simulink model "PanelsInSeriesBB_PI"  (R2016a)
settings: Solver=ode23t  StartTime=0.0  StopTime=30  FixedStep=t_PWM/10  MaxStep=2e-6  RelTol=2e-4
values from neighbouring files (symbols this model uses):
  C1 = t_PWM * (N*Impp)*0.1/ (8 * (N*Vmpp)*0.0001)    [SolarPanelModel.m]
  C2 = (N*Vo) * t_PWM/ (Load * (N*Vo)*0.001)    [SolarPanelModel.m]
  delta_Il = (N*Impp)*0.1/ 2    [SolarPanelModel.m]
  G = 1000    [SolarPanelModel.m]
  Gr = 1000    [SolarPanelModel.m]
  Isc = G/ Gr * (Iscr + miu_Isc*(Tc - Tr))    (= 9.318625)    [SolarPanelModel.m]
  Iscr = 9.19    [SolarPanelModel.m]
  K = 1.38 * 10^(-23)    (= 1.38e-23)    [SolarPanelModel.m]
  L_inductor = (N*Vo) * t_PWM/ (4 * (N*Impp)*0.01)    [SolarPanelModel.m]
  m = sol(1)    [SolarPanelModel.m]
  miu_Isc = 0.0049    [SolarPanelModel.m]
  miu_Voc = -0.1184    [SolarPanelModel.m]
  N = 3    [SolarPanelModel.m]
  NOCT = 45    [SolarPanelModel.m]
  q = 1.6 * 10^(-19)    (= 1.6e-19)    [SolarPanelModel.m]
  Rs = sol(3)    [SolarPanelModel.m]
  Rsh = sol(2)    [SolarPanelModel.m]
  T = 273.15    [SolarPanelModel.m]
  t_PWM = 20e-6    (= 2e-05)    [SolarPanelModel.m]
  ta = 20    [SolarPanelModel.m]
  Tr = T + 25    (= 298.15)    [SolarPanelModel.m]
  Vo = 50    [SolarPanelModel.m]
  Voc = Vocr + miu_Voc*(Tc - Tr) + m*Vt*log(G/Gr)    [SolarPanelModel.m]
  Vocr = 38.2    [SolarPanelModel.m]
undefined symbols (not defined in the file or in its folder): Cdc_inv, delta_Ii, g1, k2, kI, kv_ig, Li, Tpv, Tzv
libraries: powerlib x59, simulink x9, powerlib_extras x2, powerlib_meascontrol x1
settings Model: Creator=frede  LastModifiedBy=frede
settings DataIOCC: LimitDataPoints=on  SaveFormat=Array
settings HardwareCC: ProdBitPerPointer=32  ProdLargestAtomicFloat=None  ProdIntDivRoundTo=Undefined  ProdEndianess=Unspecified  ProdWordSize=32  ProdHWDeviceType=32-bit Generic
settings ModelReferenceCC: PropagateSignalLabelsOutOfModel=off
settings ConfigComp: CovModelRefEnable=Off

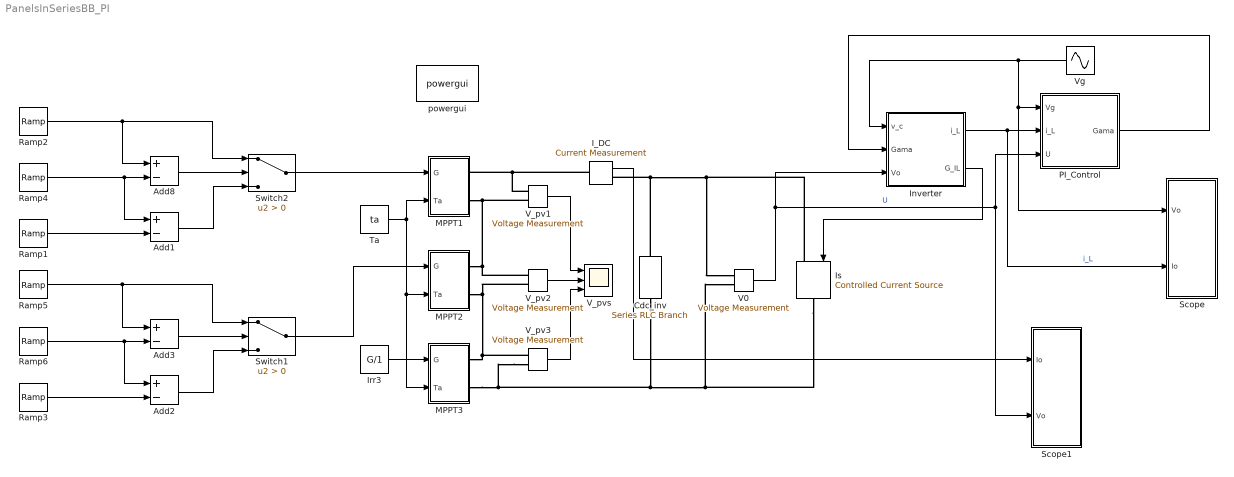
== system PanelsInSeriesBB_PI ==
  Add{1..3,8} (4 alike) : Sum  Inputs=+-
  Cdc_inv : powerlib/Elements/Series RLC Branch  LConnTagsString=__new0  RConnTagsString=__new0  BranchType=RC  Resistance=0.01  Inductance=1e-3  SetiL0=off  InitialCurrent=0  Capacitance=Cdc_inv  Setx0=on  InitialVoltage=Vo  Measurements=None
  I_DC : powerlib/Measurements/Current Measurement  PhasorSimulation=off  OutputType=Complex  PSBequivalent=0
  Inverter : Subsystem
  Irr3 : Constant  Value=G/1
  Is : powerlib/Electrical Sources/Controlled Current Source  Initialize=on  Source_Type=DC  Amplitude=0  Phase=0  Frequency=0  Measurements=None
  MPPT1 : Subsystem
  MPPT2 : Subsystem
  MPPT3 : Subsystem
  PI_Control : Subsystem
  Ramp1 : simulink/Sources/Ramp  slope=31.25  start=t5  X0=0
  Ramp2 : simulink/Sources/Ramp  slope=-31.25  start=t1  X0=g1
  Ramp3 : simulink/Sources/Ramp  slope=25  start=t6  X0=0
  Ramp4 : simulink/Sources/Ramp  slope=31.25  start=-10  X0=0
  Ramp5 : simulink/Sources/Ramp  slope=-25  start=t4  X0=g1
  Ramp6 : simulink/Sources/Ramp  slope=25  start=-20  X0=0
  Scope : Subsystem
  Scope1 : Subsystem
  Switch1 : Switch  Criteria=u2 > Threshold
  Switch2 : Switch  Criteria=u2 > Threshold
  Ta : Constant  Value=ta
  V0 : powerlib/Measurements/Voltage Measurement  PhasorSimulation=off  OutputType=Complex  PSBequivalent=0
  V_pv1 : powerlib/Measurements/Voltage Measurement  PhasorSimulation=off  OutputType=Complex  PSBequivalent=0
  V_pv2 : powerlib/Measurements/Voltage Measurement  PhasorSimulation=off  OutputType=Complex  PSBequivalent=0
  V_pv3 : powerlib/Measurements/Voltage Measurement  PhasorSimulation=off  OutputType=Complex  PSBequivalent=0
  V_pvs : Scope  NumInputPorts=3
  Vg : Sin  Amplitude=sqrt(2)*230  Frequency=2*pi*50  SampleTime=0
  powergui : powerlib/powergui  Priority=1  SimulationMode=Discrete  SolverType=Tustin/Backward Euler (TBE)  SampleTime=t_PWM/10  frequency=60  SPID=off  DisableSnubberDevices=off  DisableRonSwitches=off  DisableVfSwitches=off  SwTol=0  DisplayEquations=off  Interpol=off  ExternalGateDelay=off  methode=off  Ts=10  FunctionMessages=off  echomessages=off  HookPort=off  EnableUseOfTLC=off  x0status=blocks  frequencyindice=0  Pbase=100e6  ErrMax=1e-4  Iterations=50  UnitsV=kV  UnitsW=MW  buscounter=0  RestoreLinks=warning  ResistiveCurrentMeasurement=off  Frange=[0:2:500]  Ylog=off  Xlog=on  ShowGrid=off  save=off  variable=ZData  structure=0  ZoomFFT=off  StartTime=0.0  cycles=1  DisplayStyle=1  fundamental=60  FreqAxis=off  MaxFrequency=1000  frequencyindicesteady=1  RmsSteady=1  display=off
  wires:
  V_pv1/1 -> V_pvs/1
  V_pv2/1 -> V_pvs/2
  V_pv3/1 -> V_pvs/3
  Ta/1 -> MPPT1/2(Ta), MPPT3/2(Ta), MPPT2/2(Ta)
  Irr3/1 -> MPPT3/1(G)
  Switch2/1 -> MPPT1/1(G)
  Switch1/1 -> MPPT2/1(G)
  Vg/1 -> Inverter/1(v_c), Scope/1(Vo), PI_Control/1(Vg)
  PI_Control/1(Gama) -> Inverter/2(Gama)
  Inverter/1(i_L) -> Scope/2(Io), PI_Control/2(i_L)  "i_L"
  V0/1 -> Inverter/3(Vo), PI_Control/3(U), Scope1/2(Vo)  "U"
  Inverter/2(G_IL) -> Is/1
  I_DC/1 -> Scope1/1(Io)
  Ramp4/1 -> Add1/1, Add8/2
  Ramp2/1 -> Switch2/1, Add8/1
  Add8/1 -> Switch2/2
  Ramp1/1 -> Add1/2
  Add1/1 -> Switch2/3
  Ramp6/1 -> Add2/1, Add3/2
  Ramp5/1 -> Switch1/1, Add3/1
  Add3/1 -> Switch1/2
  Ramp3/1 -> Add2/2
  Add2/1 -> Switch1/3
  connections:
  V_pv2/LConn1 -- V_pv1/LConn2 -- MPPT1/RConn2 -- MPPT2/RConn1
  V_pv3/LConn1 -- MPPT3/RConn1 -- V_pv2/LConn2 -- MPPT2/RConn2
  I_DC/LConn1 -- V_pv1/LConn1 -- MPPT1/RConn1
  V_pv3/LConn2 -- Is/RConn1 -- V0/LConn2 -- Cdc_inv/RConn1 -- MPPT3/RConn2
  Cdc_inv/LConn1 -- Is/LConn1 -- V0/LConn1 -- I_DC/RConn1

== system PanelsInSeriesBB_PI/Inverter ==
  v_c : Inport
  Gama : Inport  Port=2
  Vo : Inport  Port=3
  Add1 : Sum  Inputs=+-
  Product : Product
  Product1 : Product
  Transfer Fcn : TransferFcn  Denominator=[Li 3]
  i_L : Outport
  G_IL : Outport  Port=2
  wires:
  Transfer Fcn/1 -> i_L/1, Product/2
  Add1/1 -> Transfer Fcn/1
  Product/1 -> G_IL/1
  Product1/1 -> Add1/1
  v_c/1 -> Add1/2
  Gama/1 -> Product1/2, Product/1
  Vo/1 -> Product1/1

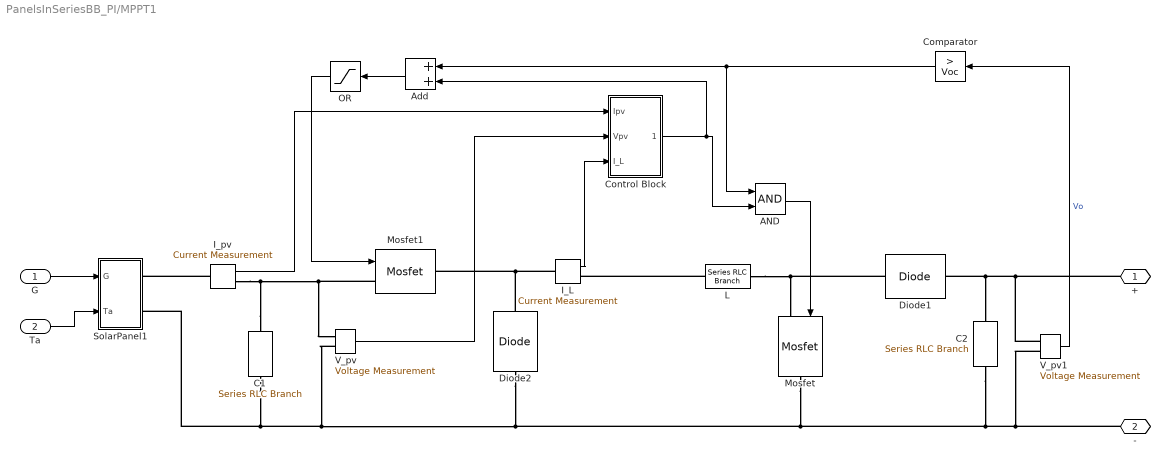
== system PanelsInSeriesBB_PI/MPPT1 ==
  G : Inport
  Ta : Inport  Port=2
  AND : Logic  AllPortsSameDT=off  OutDataTypeStr=boolean
  Add : Sum
  C1 : powerlib/Elements/Series RLC Branch  LConnTagsString=__new0  RConnTagsString=__new0  BranchType=C  Resistance=Rs  Inductance=1e-3  SetiL0=off  InitialCurrent=0  Capacitance=C1  Setx0=on  InitialVoltage=Vmpp  Measurements=None
  C2 : powerlib/Elements/Series RLC Branch  LConnTagsString=__new0  RConnTagsString=__new0  BranchType=C  Resistance=Rs  Inductance=1e-3  SetiL0=off  InitialCurrent=0  Capacitance=C2  Setx0=on  InitialVoltage=Vo/3  Measurements=None
  Comparator : simulink/Logic and Bit Operations/Compare To Constant  relop=>  const=Voc  OutDataTypeStr=boolean
  Control Block : Subsystem
  Diode1 : powerlib/Power Electronics/Diode  Ron=0.001  Lon=0  Vf=0.001  IC=0  UseSnubber=off  Rs=500  Cs=1e-9  Measurements=off
  Diode2 : powerlib/Power Electronics/Diode  Ron=0.001  Lon=0  Vf=0.001  IC=0  UseSnubber=off  Rs=500  Cs=1e-9  Measurements=off
  I_L : powerlib/Measurements/Current Measurement  PhasorSimulation=off  OutputType=Complex  PSBequivalent=0
  I_pv : powerlib/Measurements/Current Measurement  PhasorSimulation=off  OutputType=Complex  PSBequivalent=0
  L : powerlib/Elements/Series RLC Branch  LConnTagsString=__new0  RConnTagsString=__new0  BranchType=L  Resistance=Rs  Inductance=L_inductor  SetiL0=off  InitialCurrent=0  Capacitance=1e-6  Setx0=off  InitialVoltage=0  Measurements=None
  Mosfet : powerlib/Power Electronics/Mosfet  Ron=0.001  Lon=0  Rd=0.001  Vfd=0  IC=0  Rs=1e3  Cs=1e-9  Measurements=off
  Mosfet1 : powerlib/Power Electronics/Mosfet  Ron=0.001  Lon=0  Rd=0.001  Vfd=0  IC=0  Rs=1e3  Cs=1e-9  Measurements=off
  OR : Saturate  UpperLimit=1  LowerLimit=0
  SolarPanel1 : Subsystem
  V_pv : powerlib/Measurements/Voltage Measurement  PhasorSimulation=off  OutputType=Complex  PSBequivalent=0
  V_pv1 : powerlib/Measurements/Voltage Measurement  PhasorSimulation=off  OutputType=Complex  PSBequivalent=0
  + : PMIOPort  Port=1  Side=Right
  - : PMIOPort  Port=2  Side=Right
  wires:
  I_L/1 -> Control Block/3(I_L)
  Ta/1 -> SolarPanel1/2(Ta)
  G/1 -> SolarPanel1/1(G)
  V_pv1/1 -> Comparator/1  "Vo"
  Comparator/1 -> Add/1, AND/1
  Control Block/1(Gama) -> AND/2, Add/2
  Add/1 -> OR/1
  OR/1 -> Mosfet1/1
  V_pv/1 -> Control Block/2(Vpv)
  I_pv/1 -> Control Block/1(Ipv)
  AND/1 -> Mosfet/1
  connections:
  L/RConn1 -- Diode1/LConn1 -- Mosfet/LConn1
  C2/RConn1 -- Mosfet/RConn1 -- C1/RConn1 -- SolarPanel1/RConn2 -- V_pv/LConn2 -- Diode2/LConn1 -- -/RConn1 -- V_pv1/LConn2
  L/LConn1 -- I_L/RConn1
  C1/LConn1 -- I_pv/RConn1 -- Mosfet1/LConn1 -- V_pv/LConn1
  Diode2/RConn1 -- Mosfet1/RConn1 -- I_L/LConn1
  I_pv/LConn1 -- SolarPanel1/RConn1
  V_pv1/LConn1 -- +/RConn1 -- C2/LConn1 -- Diode1/RConn1

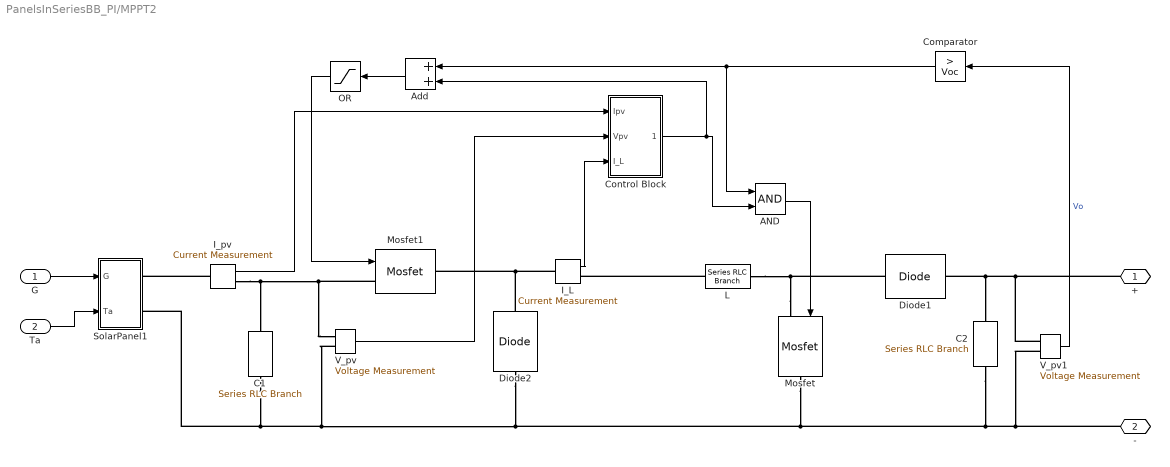
== system PanelsInSeriesBB_PI/MPPT2 ==
  G : Inport
  Ta : Inport  Port=2
  AND : Logic  AllPortsSameDT=off  OutDataTypeStr=boolean
  Add : Sum
  C1 : powerlib/Elements/Series RLC Branch  LConnTagsString=__new0  RConnTagsString=__new0  BranchType=C  Resistance=Rs  Inductance=1e-3  SetiL0=off  InitialCurrent=0  Capacitance=C1  Setx0=on  InitialVoltage=Vmpp  Measurements=None
  C2 : powerlib/Elements/Series RLC Branch  LConnTagsString=__new0  RConnTagsString=__new0  BranchType=C  Resistance=Rs  Inductance=1e-3  SetiL0=off  InitialCurrent=0  Capacitance=C2  Setx0=on  InitialVoltage=Vo/3  Measurements=None
  Comparator : simulink/Logic and Bit Operations/Compare To Constant  relop=>  const=Voc  OutDataTypeStr=boolean
  Control Block : Subsystem
  Diode1 : powerlib/Power Electronics/Diode  Ron=0.001  Lon=0  Vf=0.001  IC=0  UseSnubber=off  Rs=500  Cs=1e-9  Measurements=off
  Diode2 : powerlib/Power Electronics/Diode  Ron=0.001  Lon=0  Vf=0.001  IC=0  UseSnubber=off  Rs=500  Cs=1e-9  Measurements=off
  I_L : powerlib/Measurements/Current Measurement  PhasorSimulation=off  OutputType=Complex  PSBequivalent=0
  I_pv : powerlib/Measurements/Current Measurement  PhasorSimulation=off  OutputType=Complex  PSBequivalent=0
  L : powerlib/Elements/Series RLC Branch  LConnTagsString=__new0  RConnTagsString=__new0  BranchType=L  Resistance=Rs  Inductance=L_inductor  SetiL0=off  InitialCurrent=0  Capacitance=1e-6  Setx0=off  InitialVoltage=0  Measurements=None
  Mosfet : powerlib/Power Electronics/Mosfet  Ron=0.001  Lon=0  Rd=0.001  Vfd=0  IC=0  Rs=1e3  Cs=1e-9  Measurements=off
  Mosfet1 : powerlib/Power Electronics/Mosfet  Ron=0.001  Lon=0  Rd=0.001  Vfd=0  IC=0  Rs=1e3  Cs=1e-9  Measurements=off
  OR : Saturate  UpperLimit=1  LowerLimit=0
  SolarPanel1 : Subsystem
  V_pv : powerlib/Measurements/Voltage Measurement  PhasorSimulation=off  OutputType=Complex  PSBequivalent=0
  V_pv1 : powerlib/Measurements/Voltage Measurement  PhasorSimulation=off  OutputType=Complex  PSBequivalent=0
  + : PMIOPort  Port=1  Side=Right
  - : PMIOPort  Port=2  Side=Right
  wires:
  I_L/1 -> Control Block/3(I_L)
  Ta/1 -> SolarPanel1/2(Ta)
  G/1 -> SolarPanel1/1(G)
  V_pv1/1 -> Comparator/1  "Vo"
  Comparator/1 -> Add/1, AND/1
  Control Block/1(Gama) -> AND/2, Add/2
  Add/1 -> OR/1
  OR/1 -> Mosfet1/1
  V_pv/1 -> Control Block/2(Vpv)
  I_pv/1 -> Control Block/1(Ipv)
  AND/1 -> Mosfet/1
  connections:
  Mosfet/LConn1 -- L/RConn1 -- Diode1/LConn1
  C2/RConn1 -- Mosfet/RConn1 -- C1/RConn1 -- SolarPanel1/RConn2 -- V_pv/LConn2 -- Diode2/LConn1 -- -/RConn1 -- V_pv1/LConn2
  L/LConn1 -- I_L/RConn1
  V_pv/LConn1 -- I_pv/RConn1 -- C1/LConn1 -- Mosfet1/LConn1
  I_L/LConn1 -- Diode2/RConn1 -- Mosfet1/RConn1
  I_pv/LConn1 -- SolarPanel1/RConn1
  V_pv1/LConn1 -- +/RConn1 -- Diode1/RConn1 -- C2/LConn1

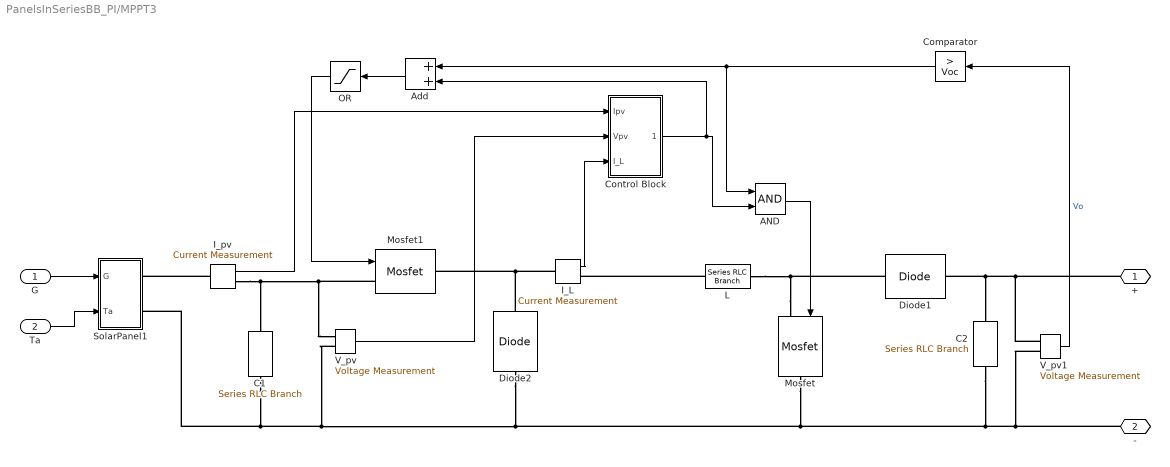
== system PanelsInSeriesBB_PI/MPPT3 ==
  G : Inport
  Ta : Inport  Port=2
  AND : Logic  AllPortsSameDT=off  OutDataTypeStr=boolean
  Add : Sum
  C1 : powerlib/Elements/Series RLC Branch  LConnTagsString=__new0  RConnTagsString=__new0  BranchType=C  Resistance=Rs  Inductance=1e-3  SetiL0=off  InitialCurrent=0  Capacitance=C1  Setx0=on  InitialVoltage=Vmpp  Measurements=None
  C2 : powerlib/Elements/Series RLC Branch  LConnTagsString=__new0  RConnTagsString=__new0  BranchType=C  Resistance=Rs  Inductance=1e-3  SetiL0=off  InitialCurrent=0  Capacitance=C2  Setx0=on  InitialVoltage=Vo/3  Measurements=None
  Comparator : simulink/Logic and Bit Operations/Compare To Constant  relop=>  const=Voc  OutDataTypeStr=boolean
  Control Block : Subsystem
  Diode1 : powerlib/Power Electronics/Diode  Ron=0.001  Lon=0  Vf=0.001  IC=0  UseSnubber=off  Rs=500  Cs=1e-9  Measurements=off
  Diode2 : powerlib/Power Electronics/Diode  Ron=0.001  Lon=0  Vf=0.001  IC=0  UseSnubber=off  Rs=500  Cs=1e-9  Measurements=off
  I_L : powerlib/Measurements/Current Measurement  PhasorSimulation=off  OutputType=Complex  PSBequivalent=0
  I_pv : powerlib/Measurements/Current Measurement  PhasorSimulation=off  OutputType=Complex  PSBequivalent=0
  L : powerlib/Elements/Series RLC Branch  LConnTagsString=__new0  RConnTagsString=__new0  BranchType=L  Resistance=Rs  Inductance=L_inductor  SetiL0=off  InitialCurrent=0  Capacitance=1e-6  Setx0=off  InitialVoltage=0  Measurements=None
  Mosfet : powerlib/Power Electronics/Mosfet  Ron=0.001  Lon=0  Rd=0.001  Vfd=0  IC=0  Rs=1e3  Cs=1e-9  Measurements=off
  Mosfet1 : powerlib/Power Electronics/Mosfet  Ron=0.001  Lon=0  Rd=0.001  Vfd=0  IC=0  Rs=1e3  Cs=1e-9  Measurements=off
  OR : Saturate  UpperLimit=1  LowerLimit=0
  SolarPanel1 : Subsystem
  V_pv : powerlib/Measurements/Voltage Measurement  PhasorSimulation=off  OutputType=Complex  PSBequivalent=0
  V_pv1 : powerlib/Measurements/Voltage Measurement  PhasorSimulation=off  OutputType=Complex  PSBequivalent=0
  + : PMIOPort  Port=1  Side=Right
  - : PMIOPort  Port=2  Side=Right
  wires:
  I_L/1 -> Control Block/3(I_L)
  Ta/1 -> SolarPanel1/2(Ta)
  G/1 -> SolarPanel1/1(G)
  V_pv1/1 -> Comparator/1  "Vo"
  Comparator/1 -> Add/1, AND/1
  Control Block/1(Gama) -> AND/2, Add/2
  Add/1 -> OR/1
  OR/1 -> Mosfet1/1
  V_pv/1 -> Control Block/2(Vpv)
  I_pv/1 -> Control Block/1(Ipv)
  AND/1 -> Mosfet/1
  connections:
  Mosfet/LConn1 -- L/RConn1 -- Diode1/LConn1
  C2/RConn1 -- Mosfet/RConn1 -- C1/RConn1 -- SolarPanel1/RConn2 -- V_pv/LConn2 -- Diode2/LConn1 -- -/RConn1 -- V_pv1/LConn2
  L/LConn1 -- I_L/RConn1
  V_pv/LConn1 -- I_pv/RConn1 -- C1/LConn1 -- Mosfet1/LConn1
  I_L/LConn1 -- Diode2/RConn1 -- Mosfet1/RConn1
  I_pv/LConn1 -- SolarPanel1/RConn1
  V_pv1/LConn1 -- +/RConn1 -- Diode1/RConn1 -- C2/LConn1

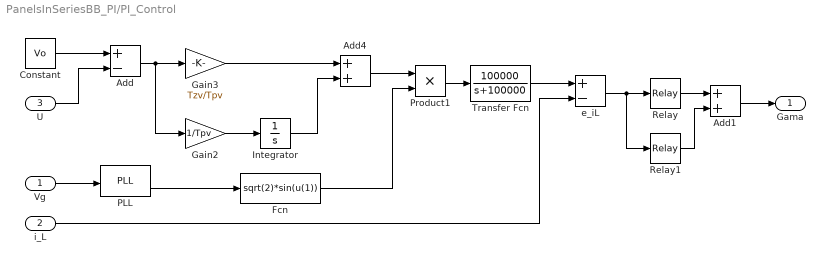
== system PanelsInSeriesBB_PI/PI_Control ==
  Vg : Inport
  i_L : Inport  Port=2
  U : Inport  Port=3
  Add : Sum  Inputs=+-
  Add1 : Sum
  Add4 : Sum
  Constant : Constant  Value=Vo
  Fcn : Fcn  Expr=sqrt(2)*sin(u(1))
  Gain2 : Gain  Gain=1/Tpv
  Gain3 : Gain  Gain=Tzv/Tpv
  Integrator : Integrator  UpperSaturationLimit=30  LowerSaturationLimit=-30  ZeroCross=off
  PLL : powerlib_meascontrol/PLL/PLL  Fmin=45  Par_Init=[0, 50]  ParK=[180, 3200, 1]  TcD=1e-4  MaxRateChangeFreq=12  FilterCutOffFreq=25  Ts=0  AGC=on
  Product1 : Product
  Relay : Relay  OnSwitchValue=delta_Ii  OffSwitchValue=-delta_Ii  OnOutputValue=0.5  OffOutputValue=-0.5  ZeroCross=off
  Relay1 : Relay  OnSwitchValue=delta_Ii/2  OffSwitchValue=-delta_Ii/2  OnOutputValue=0.5  OffOutputValue=-0.5  ZeroCross=off
  Transfer Fcn : TransferFcn  Numerator=[100000]  Denominator=[1 100000]
  e_iL : Sum  Inputs=+-
  Gama : Outport
  wires:
  Constant/1 -> Add/1
  Add/1 -> Gain2/1, Gain3/1
  U/1 -> Add/2
  Relay/1 -> Add1/1
  Relay1/1 -> Add1/2
  Add4/1 -> Product1/1
  Product1/1 -> Transfer Fcn/1
  i_L/1 -> e_iL/2
  Gain2/1 -> Integrator/1
  Gain3/1 -> Add4/1
  Integrator/1 -> Add4/2
  Add1/1 -> Gama/1
  e_iL/1 -> Relay/1, Relay1/1
  PLL/2 -> Fcn/1
  Vg/1 -> PLL/1
  Fcn/1 -> Product1/2
  Transfer Fcn/1 -> e_iL/1

== system PanelsInSeriesBB_PI/Scope ==
  Vo : Inport
  Io : Inport  Port=2
  Grid : Scope  NumInputPorts=3
  P_o : Subsystem
  To Workspace : ToWorkspace  VariableName=Pg  SaveFormat=Timeseries  SampleTime=-1
  wires:
  P_o/1(P) -> To Workspace/1, Grid/3
  Io/1 -> Grid/2, P_o/2(i)
  Vo/1 -> Grid/1, P_o/1(v)

== system PanelsInSeriesBB_PI/Scope1 ==
  Io : Inport
  Vo : Inport  Port=2
  DC side : Scope  NumInputPorts=3
  P_o : Subsystem
  To Workspace : ToWorkspace  VariableName=Po  SaveFormat=Timeseries  SampleTime=-1
  To Workspace1 : ToWorkspace  VariableName=Vo  SaveFormat=Timeseries  SampleTime=-1
  wires:
  P_o/1(P) -> To Workspace/1, DC side/3
  Io/1 -> DC side/2, P_o/2(i)
  Vo/1 -> To Workspace1/1, DC side/1, P_o/1(v)

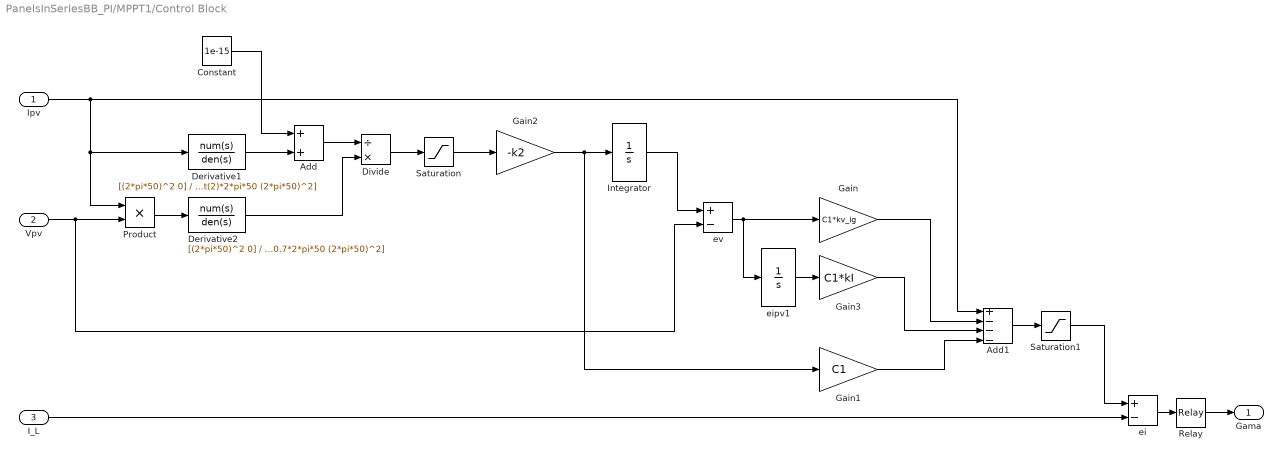
== system PanelsInSeriesBB_PI/MPPT1/Control Block ==
  Ipv : Inport
  Vpv : Inport  Port=2
  I_L : Inport  Port=3
  Add : Sum
  Add1 : Sum  Inputs=+---
  Constant : Constant  Value=1e-15
  Derivative1 : TransferFcn  Numerator=[(2*pi*50)^2 0]  Denominator=[1 sqrt(2)*2*pi*50 (2*pi*50)^2]
  Derivative2 : TransferFcn  Numerator=[(2*pi*50)^2 0]  Denominator=[1 sqrt(2)*0.7*2*pi*50 (2*pi*50)^2]
  Divide : Product  Inputs=/*
  Gain : Gain  Gain=C1*kv_ig
  Gain1 : Gain  Gain=C1
  Gain2 : Gain  Gain=-k2
  Gain3 : Gain  Gain=C1*kI
  Integrator : Integrator  InitialCondition=Voc*0.75  LimitOutput=on  UpperSaturationLimit=Voc  LowerSaturationLimit=0
  Product : Product  Inputs=**
  Relay : Relay  OnSwitchValue=delta_Il  OffSwitchValue=-delta_Il
  Saturation : Saturate  UpperLimit=2  LowerLimit=-2
  Saturation1 : Saturate  UpperLimit=Isc*1.2  LowerLimit=0
  ei : Sum  Inputs=+-
  eipv1 : Integrator  UpperSaturationLimit=Voc*N  LowerSaturationLimit=0
  ev : Sum  Inputs=+-
  Gama : Outport
  wires:
  ev/1 -> eipv1/1, Gain/1
  Gain/1 -> Add1/2
  Gain1/1 -> Add1/4
  Integrator/1 -> ev/1
  eipv1/1 -> Gain3/1
  Gain3/1 -> Add1/3
  Add1/1 -> Saturation1/1
  I_L/1 -> ei/2
  ei/1 -> Relay/1
  Relay/1 -> Gama/1
  Saturation1/1 -> ei/1
  Saturation/1 -> Gain2/1
  Derivative1/1 -> Add/2
  Constant/1 -> Add/1
  Gain2/1 -> Integrator/1, Gain1/1
  Product/1 -> Derivative2/1
  Divide/1 -> Saturation/1
  Add/1 -> Divide/1
  Derivative2/1 -> Divide/2
  Ipv/1 -> Add1/1, Derivative1/1, Product/1
  Vpv/1 -> ev/2, Product/2

== system PanelsInSeriesBB_PI/MPPT1/SolarPanel1 ==
  G : Inport
  Ta : Inport  Port=2
  Diode : Subsystem  AncestorBlock=re_lib/Solar/PV Array/Diode Rsh
      mask Display:
      | plot(-75,-50,100,150, [-15 -15 43 -15 -15 -75],[50 8 50 92 50 50], ...
      |     [43 43],[8 94],[100 43], [50 50])
  Diode1 : powerlib/Power Electronics/Diode  Ron=0.001  Lon=0  Vf=0  IC=0  UseSnubber=off  Rs=500  Cs=250e-9  Measurements=off
  Ev.Conditions : Subsystem
  Is : powerlib/Electrical Sources/Controlled Current Source  Initialize=on  Source_Type=DC  Amplitude=0  Phase=0  Frequency=0  Measurements=None
  Rs : powerlib/Elements/Series RLC Branch  LConnTagsString=__new0  RConnTagsString=__new0  BranchType=R  Resistance=Rs  Inductance=1e-3  SetiL0=off  InitialCurrent=0  Capacitance=1e-6  Setx0=off  InitialVoltage=0  Measurements=None
  Rsh : powerlib/Elements/Series RLC Branch  LConnTagsString=__new0  RConnTagsString=__new0  BranchType=R  Resistance=Rsh  Inductance=1e-3  SetiL0=off  InitialCurrent=0  Capacitance=1e-6  Setx0=off  InitialVoltage=0  Measurements=None
  + : PMIOPort  Port=1  Side=Right
  - : PMIOPort  Port=2  Side=Right
  wires:
  G/1 -> Ev.Conditions/1(G)
  Ta/1 -> Ev.Conditions/2(Ta)
  Ev.Conditions/2(Io) -> Diode/1(Io)
  Ev.Conditions/1(Vt) -> Diode/2(Vt)
  Ev.Conditions/3(Is) -> Is/1
  connections:
  Is/RConn1 -- Diode/LConn1 -- Rsh/LConn1 -- Rs/LConn1
  Rsh/RConn1 -- -/RConn1 -- Diode1/LConn1 -- Is/LConn1 -- Diode/RConn1
  Diode1/RConn1 -- +/RConn1 -- Rs/RConn1

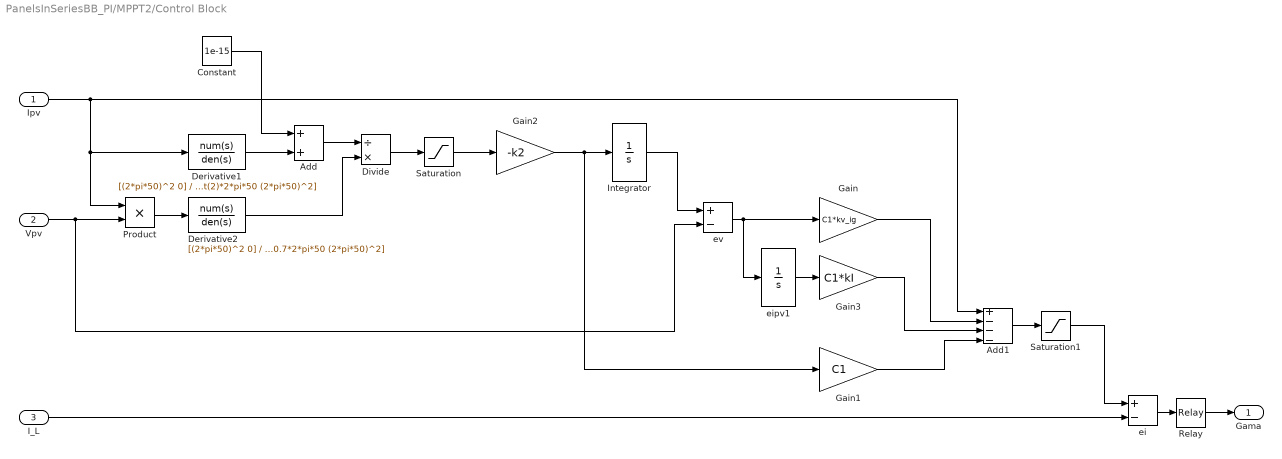
== system PanelsInSeriesBB_PI/MPPT2/Control Block ==
  Ipv : Inport
  Vpv : Inport  Port=2
  I_L : Inport  Port=3
  Add : Sum
  Add1 : Sum  Inputs=+---
  Constant : Constant  Value=1e-15
  Derivative1 : TransferFcn  Numerator=[(2*pi*50)^2 0]  Denominator=[1 sqrt(2)*2*pi*50 (2*pi*50)^2]
  Derivative2 : TransferFcn  Numerator=[(2*pi*50)^2 0]  Denominator=[1 sqrt(2)*0.7*2*pi*50 (2*pi*50)^2]
  Divide : Product  Inputs=/*
  Gain : Gain  Gain=C1*kv_ig
  Gain1 : Gain  Gain=C1
  Gain2 : Gain  Gain=-k2
  Gain3 : Gain  Gain=C1*kI
  Integrator : Integrator  InitialCondition=Voc*0.75  LimitOutput=on  UpperSaturationLimit=Voc  LowerSaturationLimit=0
  Product : Product  Inputs=**
  Relay : Relay  OnSwitchValue=delta_Il  OffSwitchValue=-delta_Il
  Saturation : Saturate  UpperLimit=2  LowerLimit=-2
  Saturation1 : Saturate  UpperLimit=Isc*1.2  LowerLimit=0
  ei : Sum  Inputs=+-
  eipv1 : Integrator  UpperSaturationLimit=Voc*N  LowerSaturationLimit=0
  ev : Sum  Inputs=+-
  Gama : Outport
  wires:
  ev/1 -> eipv1/1, Gain/1
  Gain/1 -> Add1/2
  Gain1/1 -> Add1/4
  Integrator/1 -> ev/1
  eipv1/1 -> Gain3/1
  Gain3/1 -> Add1/3
  Add1/1 -> Saturation1/1
  I_L/1 -> ei/2
  ei/1 -> Relay/1
  Relay/1 -> Gama/1
  Saturation1/1 -> ei/1
  Saturation/1 -> Gain2/1
  Derivative1/1 -> Add/2
  Constant/1 -> Add/1
  Gain2/1 -> Integrator/1, Gain1/1
  Product/1 -> Derivative2/1
  Divide/1 -> Saturation/1
  Add/1 -> Divide/1
  Derivative2/1 -> Divide/2
  Ipv/1 -> Add1/1, Derivative1/1, Product/1
  Vpv/1 -> ev/2, Product/2

== system PanelsInSeriesBB_PI/MPPT2/SolarPanel1 ==
  G : Inport
  Ta : Inport  Port=2
  Diode : Subsystem  AncestorBlock=re_lib/Solar/PV Array/Diode Rsh
      mask Display:
      | plot(-75,-50,100,150, [-15 -15 43 -15 -15 -75],[50 8 50 92 50 50], ...
      |     [43 43],[8 94],[100 43], [50 50])
  Diode1 : powerlib/Power Electronics/Diode  Ron=0.001  Lon=0  Vf=0  IC=0  UseSnubber=off  Rs=500  Cs=250e-9  Measurements=off
  Ev.Conditions : Subsystem
  Is : powerlib/Electrical Sources/Controlled Current Source  Initialize=on  Source_Type=DC  Amplitude=0  Phase=0  Frequency=0  Measurements=None
  Rs : powerlib/Elements/Series RLC Branch  LConnTagsString=__new0  RConnTagsString=__new0  BranchType=R  Resistance=Rs  Inductance=1e-3  SetiL0=off  InitialCurrent=0  Capacitance=1e-6  Setx0=off  InitialVoltage=0  Measurements=None
  Rsh : powerlib/Elements/Series RLC Branch  LConnTagsString=__new0  RConnTagsString=__new0  BranchType=R  Resistance=Rsh  Inductance=1e-3  SetiL0=off  InitialCurrent=0  Capacitance=1e-6  Setx0=off  InitialVoltage=0  Measurements=None
  + : PMIOPort  Port=1  Side=Right
  - : PMIOPort  Port=2  Side=Right
  wires:
  G/1 -> Ev.Conditions/1(G)
  Ta/1 -> Ev.Conditions/2(Ta)
  Ev.Conditions/2(Io) -> Diode/1(Io)
  Ev.Conditions/1(Vt) -> Diode/2(Vt)
  Ev.Conditions/3(Is) -> Is/1
  connections:
  Rsh/LConn1 -- Rs/LConn1 -- Is/RConn1 -- Diode/LConn1
  Rsh/RConn1 -- -/RConn1 -- Diode1/LConn1 -- Is/LConn1 -- Diode/RConn1
  Diode1/RConn1 -- +/RConn1 -- Rs/RConn1

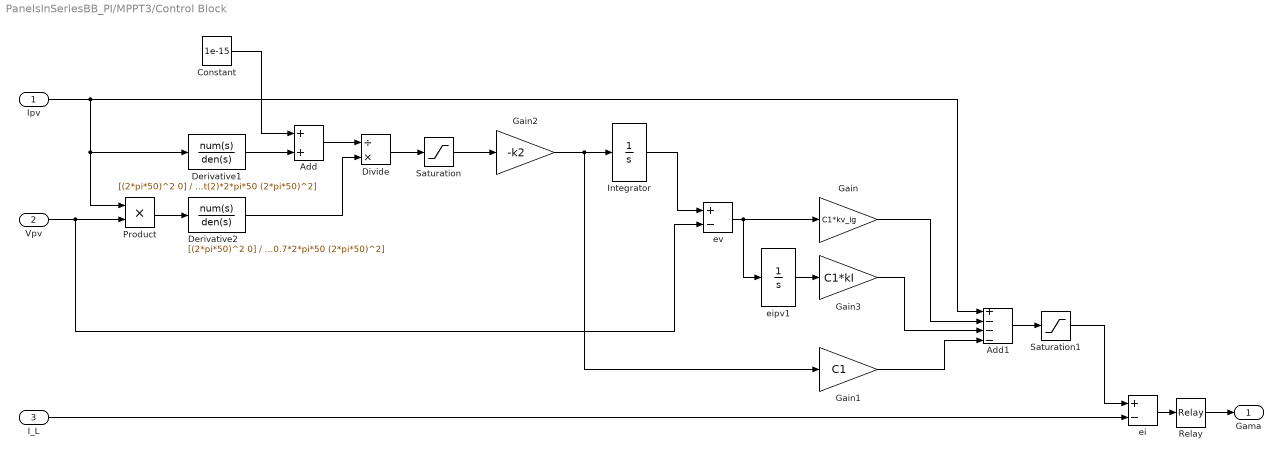
== system PanelsInSeriesBB_PI/MPPT3/Control Block ==
  Ipv : Inport
  Vpv : Inport  Port=2
  I_L : Inport  Port=3
  Add : Sum
  Add1 : Sum  Inputs=+---
  Constant : Constant  Value=1e-15
  Derivative1 : TransferFcn  Numerator=[(2*pi*50)^2 0]  Denominator=[1 sqrt(2)*2*pi*50 (2*pi*50)^2]
  Derivative2 : TransferFcn  Numerator=[(2*pi*50)^2 0]  Denominator=[1 sqrt(2)*0.7*2*pi*50 (2*pi*50)^2]
  Divide : Product  Inputs=/*
  Gain : Gain  Gain=C1*kv_ig
  Gain1 : Gain  Gain=C1
  Gain2 : Gain  Gain=-k2
  Gain3 : Gain  Gain=C1*kI
  Integrator : Integrator  InitialCondition=Voc*0.75  LimitOutput=on  UpperSaturationLimit=Voc  LowerSaturationLimit=0
  Product : Product  Inputs=**
  Relay : Relay  OnSwitchValue=delta_Il  OffSwitchValue=-delta_Il
  Saturation : Saturate  UpperLimit=2  LowerLimit=-2
  Saturation1 : Saturate  UpperLimit=Isc*1.2  LowerLimit=0
  ei : Sum  Inputs=+-
  eipv1 : Integrator  UpperSaturationLimit=Voc*N  LowerSaturationLimit=0
  ev : Sum  Inputs=+-
  Gama : Outport
  wires:
  ev/1 -> eipv1/1, Gain/1
  Gain/1 -> Add1/2
  Gain1/1 -> Add1/4
  Integrator/1 -> ev/1
  eipv1/1 -> Gain3/1
  Gain3/1 -> Add1/3
  Add1/1 -> Saturation1/1
  I_L/1 -> ei/2
  ei/1 -> Relay/1
  Relay/1 -> Gama/1
  Saturation1/1 -> ei/1
  Saturation/1 -> Gain2/1
  Derivative1/1 -> Add/2
  Constant/1 -> Add/1
  Gain2/1 -> Integrator/1, Gain1/1
  Product/1 -> Derivative2/1
  Divide/1 -> Saturation/1
  Add/1 -> Divide/1
  Derivative2/1 -> Divide/2
  Ipv/1 -> Add1/1, Derivative1/1, Product/1
  Vpv/1 -> ev/2, Product/2

== system PanelsInSeriesBB_PI/MPPT3/SolarPanel1 ==
  G : Inport
  Ta : Inport  Port=2
  Diode : Subsystem  AncestorBlock=re_lib/Solar/PV Array/Diode Rsh
      mask Display:
      | plot(-75,-50,100,150, [-15 -15 43 -15 -15 -75],[50 8 50 92 50 50], ...
      |     [43 43],[8 94],[100 43], [50 50])
  Diode1 : powerlib/Power Electronics/Diode  Ron=0.001  Lon=0  Vf=0  IC=0  UseSnubber=off  Rs=500  Cs=250e-9  Measurements=off
  Ev.Conditions : Subsystem
  Is : powerlib/Electrical Sources/Controlled Current Source  Initialize=on  Source_Type=DC  Amplitude=0  Phase=0  Frequency=0  Measurements=None
  Rs : powerlib/Elements/Series RLC Branch  LConnTagsString=__new0  RConnTagsString=__new0  BranchType=R  Resistance=Rs  Inductance=1e-3  SetiL0=off  InitialCurrent=0  Capacitance=1e-6  Setx0=off  InitialVoltage=0  Measurements=None
  Rsh : powerlib/Elements/Series RLC Branch  LConnTagsString=__new0  RConnTagsString=__new0  BranchType=R  Resistance=Rsh  Inductance=1e-3  SetiL0=off  InitialCurrent=0  Capacitance=1e-6  Setx0=off  InitialVoltage=0  Measurements=None
  + : PMIOPort  Port=1  Side=Right
  - : PMIOPort  Port=2  Side=Right
  wires:
  G/1 -> Ev.Conditions/1(G)
  Ta/1 -> Ev.Conditions/2(Ta)
  Ev.Conditions/2(Io) -> Diode/1(Io)
  Ev.Conditions/1(Vt) -> Diode/2(Vt)
  Ev.Conditions/3(Is) -> Is/1
  connections:
  Rsh/LConn1 -- Rs/LConn1 -- Is/RConn1 -- Diode/LConn1
  Rsh/RConn1 -- -/RConn1 -- Diode1/LConn1 -- Is/LConn1 -- Diode/RConn1
  Diode1/RConn1 -- +/RConn1 -- Rs/RConn1

== system PanelsInSeriesBB_PI/Scope/P_o ==
  v : Inport
  i : Inport  Port=2
  Mean Value : powerlib_extras/Measurements/Mean Value  Period=1/50
  Product : Product
  P : Outport
  wires:
  Mean Value/1 -> P/1
  Product/1 -> Mean Value/1
  v/1 -> Product/1
  i/1 -> Product/2

== system PanelsInSeriesBB_PI/Scope1/P_o ==
  v : Inport
  i : Inport  Port=2
  Mean Value : powerlib_extras/Measurements/Mean Value  Period=1/50
  Product : Product
  P : Outport
  wires:
  Mean Value/1 -> P/1
  Product/1 -> Mean Value/1
  v/1 -> Product/1
  i/1 -> Product/2

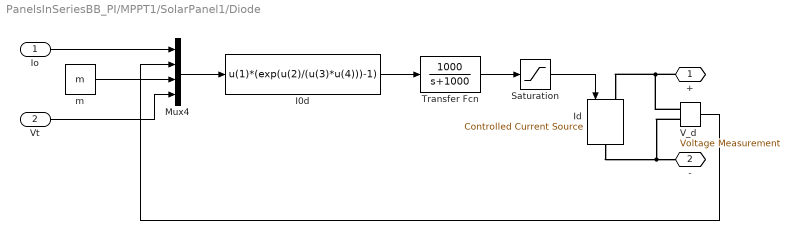
== system PanelsInSeriesBB_PI/MPPT1/SolarPanel1/Diode ==
  Io : Inport
  Vt : Inport  Port=2
  I0d : Fcn  Expr=u(1)*(exp(u(2)/(u(3)*u(4)))-1)
  Id : powerlib/Electrical Sources/Controlled Current Source  Initialize=on  Source_Type=DC  Amplitude=0  Phase=0  Frequency=0  Measurements=None
  Mux4 : Mux
  Saturation : Saturate  UpperLimit=Isc  LowerLimit=0
  Transfer Fcn : TransferFcn  Numerator=[1000]  Denominator=[1 1000]
  V_d : powerlib/Measurements/Voltage Measurement  PhasorSimulation=off  OutputType=Complex  PSBequivalent=0
  m : Constant  Value=m
  + : PMIOPort  Port=1  Side=Left
  - : PMIOPort  Port=2  Side=Right
  wires:
  Mux4/1 -> I0d/1
  Io/1 -> Mux4/1
  V_d/1 -> Mux4/2
  m/1 -> Mux4/3
  Vt/1 -> Mux4/4
  I0d/1 -> Transfer Fcn/1
  Transfer Fcn/1 -> Saturation/1
  Saturation/1 -> Id/1
  connections:
  Id/RConn1 -- V_d/LConn2 -- -/RConn1
  +/RConn1 -- V_d/LConn1 -- Id/LConn1

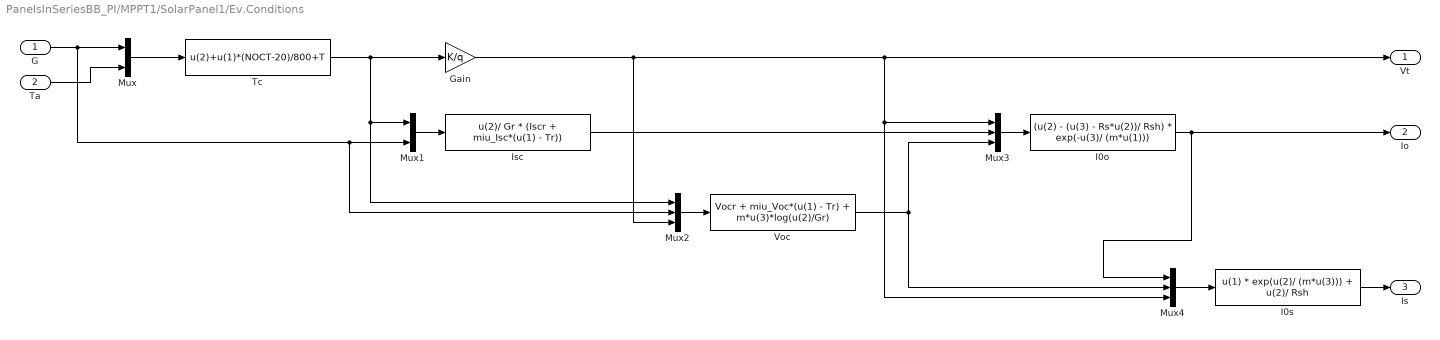
== system PanelsInSeriesBB_PI/MPPT1/SolarPanel1/Ev.Conditions ==
  G : Inport
  Ta : Inport  Port=2
  Gain : Gain  Gain=K/q
  I0o : Fcn  Expr=(u(2) - (u(3) - Rs*u(2))/ Rsh) * exp(-u(3)/ (m*u(1)))
  I0s : Fcn  Expr=u(1) * exp(u(2)/ (m*u(3))) + u(2)/ Rsh
  Isc : Fcn  Expr=u(2)/ Gr * (Iscr + miu_Isc*(u(1) - Tr))
  Mux : Mux  Inputs=2
  Mux1 : Mux  Inputs=2
  Mux2 : Mux  Inputs=3
  Mux3 : Mux  Inputs=3
  Mux4 : Mux  Inputs=3
  Tc : Fcn  Expr=u(2)+u(1)*(NOCT-20)/800+T
  Voc : Fcn  Expr=Vocr + miu_Voc*(u(1) - Tr) + m*u(3)*log(u(2)/Gr)
  Vt : Outport
  Io : Outport  Port=2
  Is : Outport  Port=3
  wires:
  Mux1/1 -> Isc/1
  Gain/1 -> Mux2/3, Vt/1, Mux4/3, Mux3/1
  Mux/1 -> Tc/1
  I0s/1 -> Is/1
  Ta/1 -> Mux/2
  G/1 -> Mux/1, Mux2/2, Mux1/2
  Tc/1 -> Mux2/1, Mux1/1, Gain/1
  I0o/1 -> Mux4/1, Io/1
  Mux2/1 -> Voc/1
  Mux3/1 -> I0o/1
  Isc/1 -> Mux3/2
  Voc/1 -> Mux3/3, Mux4/2
  Mux4/1 -> I0s/1

== system PanelsInSeriesBB_PI/MPPT2/SolarPanel1/Diode ==
  Io : Inport
  Vt : Inport  Port=2
  I0d : Fcn  Expr=u(1)*(exp(u(2)/(u(3)*u(4)))-1)
  Id : powerlib/Electrical Sources/Controlled Current Source  Initialize=on  Source_Type=DC  Amplitude=0  Phase=0  Frequency=0  Measurements=None
  Mux4 : Mux
  Saturation : Saturate  UpperLimit=Isc  LowerLimit=0
  Transfer Fcn : TransferFcn  Numerator=[1000]  Denominator=[1 1000]
  V_d : powerlib/Measurements/Voltage Measurement  PhasorSimulation=off  OutputType=Complex  PSBequivalent=0
  m : Constant  Value=m
  + : PMIOPort  Port=1  Side=Left
  - : PMIOPort  Port=2  Side=Right
  wires:
  Mux4/1 -> I0d/1
  Io/1 -> Mux4/1
  V_d/1 -> Mux4/2
  m/1 -> Mux4/3
  Vt/1 -> Mux4/4
  I0d/1 -> Transfer Fcn/1
  Transfer Fcn/1 -> Saturation/1
  Saturation/1 -> Id/1
  connections:
  Id/RConn1 -- V_d/LConn2 -- -/RConn1
  +/RConn1 -- V_d/LConn1 -- Id/LConn1

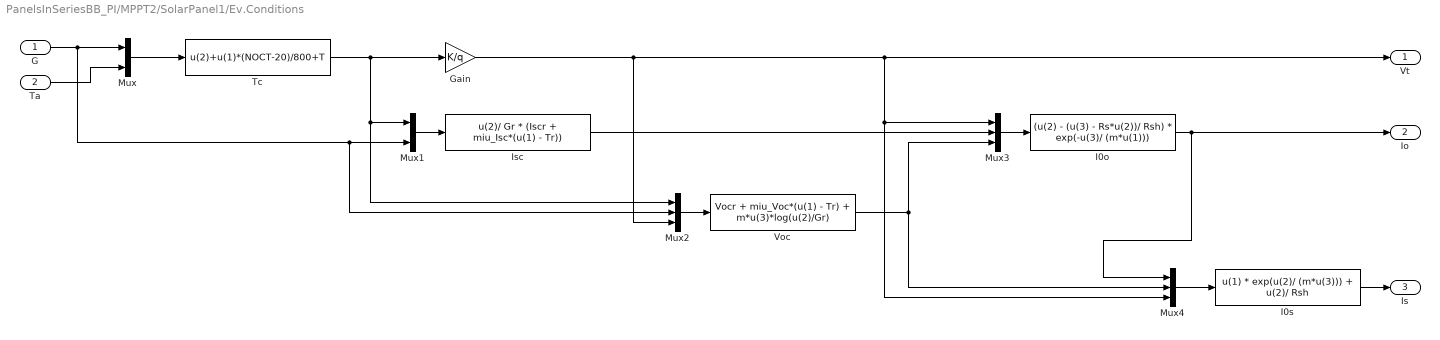
== system PanelsInSeriesBB_PI/MPPT2/SolarPanel1/Ev.Conditions ==
  G : Inport
  Ta : Inport  Port=2
  Gain : Gain  Gain=K/q
  I0o : Fcn  Expr=(u(2) - (u(3) - Rs*u(2))/ Rsh) * exp(-u(3)/ (m*u(1)))
  I0s : Fcn  Expr=u(1) * exp(u(2)/ (m*u(3))) + u(2)/ Rsh
  Isc : Fcn  Expr=u(2)/ Gr * (Iscr + miu_Isc*(u(1) - Tr))
  Mux : Mux  Inputs=2
  Mux1 : Mux  Inputs=2
  Mux2 : Mux  Inputs=3
  Mux3 : Mux  Inputs=3
  Mux4 : Mux  Inputs=3
  Tc : Fcn  Expr=u(2)+u(1)*(NOCT-20)/800+T
  Voc : Fcn  Expr=Vocr + miu_Voc*(u(1) - Tr) + m*u(3)*log(u(2)/Gr)
  Vt : Outport
  Io : Outport  Port=2
  Is : Outport  Port=3
  wires:
  Mux1/1 -> Isc/1
  Gain/1 -> Mux2/3, Vt/1, Mux4/3, Mux3/1
  Mux/1 -> Tc/1
  I0s/1 -> Is/1
  Ta/1 -> Mux/2
  G/1 -> Mux/1, Mux2/2, Mux1/2
  Tc/1 -> Mux2/1, Mux1/1, Gain/1
  I0o/1 -> Mux4/1, Io/1
  Mux2/1 -> Voc/1
  Mux3/1 -> I0o/1
  Isc/1 -> Mux3/2
  Voc/1 -> Mux3/3, Mux4/2
  Mux4/1 -> I0s/1

== system PanelsInSeriesBB_PI/MPPT3/SolarPanel1/Diode ==
  Io : Inport
  Vt : Inport  Port=2
  I0d : Fcn  Expr=u(1)*(exp(u(2)/(u(3)*u(4)))-1)
  Id : powerlib/Electrical Sources/Controlled Current Source  Initialize=on  Source_Type=DC  Amplitude=0  Phase=0  Frequency=0  Measurements=None
  Mux4 : Mux
  Saturation : Saturate  UpperLimit=Isc  LowerLimit=0
  Transfer Fcn : TransferFcn  Numerator=[1000]  Denominator=[1 1000]
  V_d : powerlib/Measurements/Voltage Measurement  PhasorSimulation=off  OutputType=Complex  PSBequivalent=0
  m : Constant  Value=m
  + : PMIOPort  Port=1  Side=Left
  - : PMIOPort  Port=2  Side=Right
  wires:
  Mux4/1 -> I0d/1
  Io/1 -> Mux4/1
  V_d/1 -> Mux4/2
  m/1 -> Mux4/3
  Vt/1 -> Mux4/4
  I0d/1 -> Transfer Fcn/1
  Transfer Fcn/1 -> Saturation/1
  Saturation/1 -> Id/1
  connections:
  Id/RConn1 -- V_d/LConn2 -- -/RConn1
  +/RConn1 -- V_d/LConn1 -- Id/LConn1

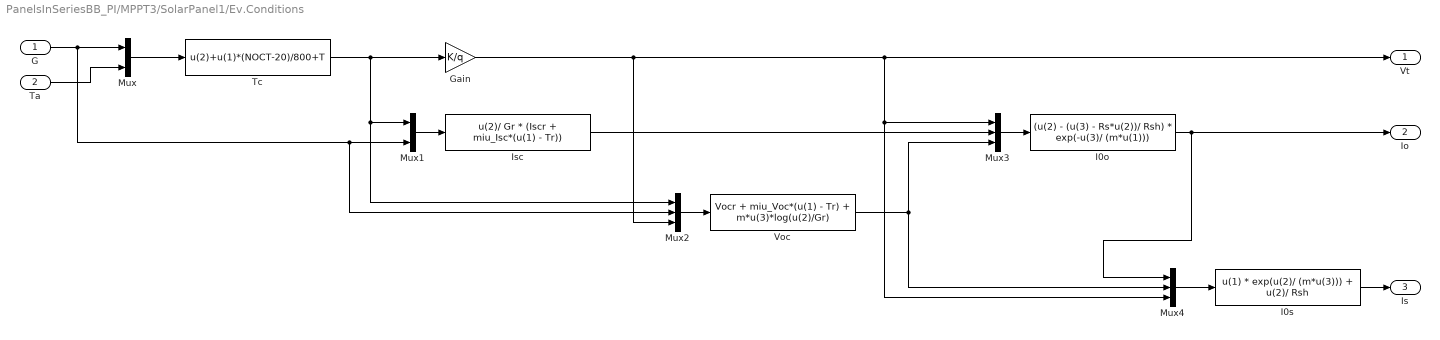
== system PanelsInSeriesBB_PI/MPPT3/SolarPanel1/Ev.Conditions ==
  G : Inport
  Ta : Inport  Port=2
  Gain : Gain  Gain=K/q
  I0o : Fcn  Expr=(u(2) - (u(3) - Rs*u(2))/ Rsh) * exp(-u(3)/ (m*u(1)))
  I0s : Fcn  Expr=u(1) * exp(u(2)/ (m*u(3))) + u(2)/ Rsh
  Isc : Fcn  Expr=u(2)/ Gr * (Iscr + miu_Isc*(u(1) - Tr))
  Mux : Mux  Inputs=2
  Mux1 : Mux  Inputs=2
  Mux2 : Mux  Inputs=3
  Mux3 : Mux  Inputs=3
  Mux4 : Mux  Inputs=3
  Tc : Fcn  Expr=u(2)+u(1)*(NOCT-20)/800+T
  Voc : Fcn  Expr=Vocr + miu_Voc*(u(1) - Tr) + m*u(3)*log(u(2)/Gr)
  Vt : Outport
  Io : Outport  Port=2
  Is : Outport  Port=3
  wires:
  Mux1/1 -> Isc/1
  Gain/1 -> Mux2/3, Vt/1, Mux4/3, Mux3/1
  Mux/1 -> Tc/1
  I0s/1 -> Is/1
  Ta/1 -> Mux/2
  G/1 -> Mux/1, Mux2/2, Mux1/2
  Tc/1 -> Mux2/1, Mux1/1, Gain/1
  I0o/1 -> Mux4/1, Io/1
  Mux2/1 -> Voc/1
  Mux3/1 -> I0o/1
  Isc/1 -> Mux3/2
  Voc/1 -> Mux3/3, Mux4/2
  Mux4/1 -> I0s/1
